simulink model "slb_multirate"  (R2015b)
settings: Solver=FixedStepDiscrete  SolverMode=SingleTasking  StartTime=0.0  StopTime=1  RelTol=1e-3
libraries: simulink x1, dspsigops x1
settings Model: Creator=at-mt  LastModifiedBy=amatsumo
settings DataIOCC: SaveFormat=Array  SignalLoggingSaveFormat=ModelDataLogs  SaveOutput=off  SignalLogging=off  SaveTime=off
settings OptimizationCC: BlockReduction=off  ConditionallyExecuteInputs=off  DefaultParameterBehavior=Inlined  ExpressionDepthLimit=2147483647
settings DebuggingCC: AlgebraicLoopMsg=error  UnderspecifiedInitializationDetection=Classic  MergeDetectMultiDrivingBlocksExec=none  SolverPrmCheckMsg=warning  SingleTaskRateTransMsg=error  FcnCallInpInsideContextMsg=UseLocalSettings  StateNameClashWarn=warning
settings HardwareCC: ProdBitPerPointer=32  ProdLargestAtomicFloat=None  ProdIntDivRoundTo=Undefined  ProdEndianess=Unspecified  ProdWordSize=32  ProdHWDeviceType=ASIC/FPGA->ASIC/FPGA  ProdEqTarget=off
settings SFSimCC: SFSimEcho=off  SimParseCustomCode=off
settings GRTTargetCC: GeneratePreprocessorConditionals=Disable all  CombineOutputUpdateFcns=off  GRTInterface=on
settings ConfigComp: CovModelRefEnable=Off  CovSFcnEnable=off

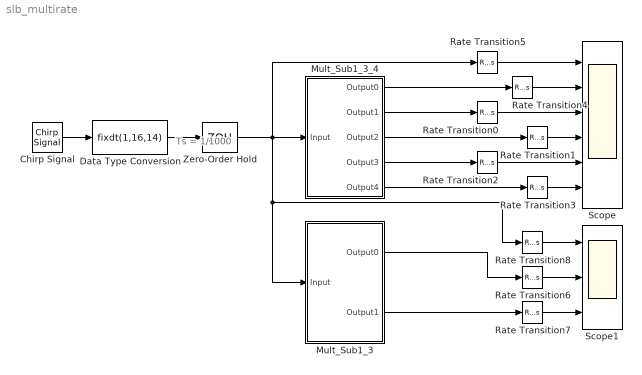
== system slb_multirate ==
  note: Ts = 1/1000
  Chirp Signal : simulink/Sources/Chirp Signal  f1=10  T=1  f2=100
  Data Type Conversion : DataTypeConversion  OutDataTypeStr=fixdt(1,16,14)
  Mult_Sub1_3 : Subsystem  Tag=FilterWizardSubSystem
      settings: ErrorFcn=dspFilterRealizedInBasicElemsAlgLoopErrFcnCallback
  Mult_Sub1_3_4 : Subsystem  Tag=FilterWizardSubSystem
      settings: ErrorFcn=dspFilterRealizedInBasicElemsAlgLoopErrFcnCallback
  Rate Transition{0..8} (9 alike) : RateTransition
  Scope : Scope  NumInputPorts=6
  Scope1 : Scope  NumInputPorts=3
  Zero-Order Hold : ZeroOrderHold  SampleTime=1/1000
  wires:
  Chirp Signal/1 -> Data Type Conversion/1
  Zero-Order Hold/1 -> Mult_Sub1_3_4/1(Input), Rate Transition5/1, Mult_Sub1_3/1(Input), Rate Transition8/1
  Data Type Conversion/1 -> Zero-Order Hold/1
  Mult_Sub1_3_4/1(Output0) -> Rate Transition4/1
  Mult_Sub1_3_4/2(Output1) -> Rate Transition0/1
  Mult_Sub1_3_4/3(Output2) -> Rate Transition1/1
  Rate Transition0/1 -> Scope/3
  Rate Transition1/1 -> Scope/4
  Mult_Sub1_3_4/4(Output3) -> Rate Transition2/1
  Mult_Sub1_3_4/5(Output4) -> Rate Transition3/1
  Rate Transition2/1 -> Scope/5
  Rate Transition3/1 -> Scope/6
  Rate Transition4/1 -> Scope/2
  Rate Transition5/1 -> Scope/1
  Mult_Sub1_3/1(Output0) -> Rate Transition6/1
  Mult_Sub1_3/2(Output1) -> Rate Transition7/1
  Rate Transition6/1 -> Scope1/2
  Rate Transition7/1 -> Scope1/3
  Rate Transition8/1 -> Scope1/1

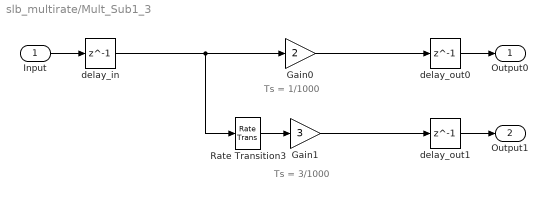
== system slb_multirate/Mult_Sub1_3 ==
  note: Ts = 1/1000
  note: Ts = 3/1000
  Input : Inport
  Gain0 : Gain  Gain=2
  Gain1 : Gain  Gain=3
  Rate Transition3 : RateTransition  OutPortSampleTime=3/1000
  delay_in : Delay  DelayLength=1  InitialCondition=0  InputProcessing=Inherited
  delay_out0 : Delay  DelayLength=1  InitialCondition=0  InputProcessing=Inherited
  delay_out1 : Delay  DelayLength=1  InitialCondition=0  InputProcessing=Inherited
  Output0 : Outport
  Output1 : Outport  Port=2
  wires:
  Gain1/1 -> delay_out1/1
  Gain0/1 -> delay_out0/1
  delay_out1/1 -> Output1/1
  Rate Transition3/1 -> Gain1/1
  delay_out0/1 -> Output0/1
  delay_in/1 -> Gain0/1, Rate Transition3/1
  Input/1 -> delay_in/1

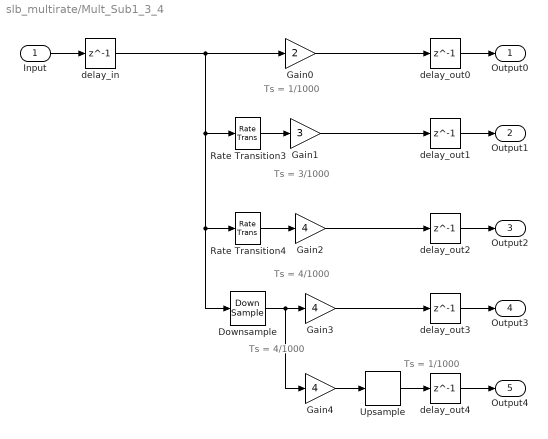
== system slb_multirate/Mult_Sub1_3_4 ==
  note: Ts = 3/1000
  note: Ts = 4/1000
  note: Ts = 1/1000
  note: Ts = 4/1000
  note: Ts = 1/1000
  Input : Inport
  Downsample : DownSample  N=4  RateOptions=Allow multirate processing
  Gain0 : Gain  Gain=2
  Gain1 : Gain  Gain=3
  Gain2 : Gain  Gain=4
  Gain3 : Gain  Gain=4
  Gain4 : Gain  Gain=4
  Rate Transition3 : RateTransition  OutPortSampleTime=3/1000
  Rate Transition4 : RateTransition  OutPortSampleTime=4/1000
  Upsample : dspsigops/Upsample  N=4  phase=0  InputProcessing=Columns as channels (frame based)  RateOptions=Allow multirate processing  ic=0  mode=Unused parameter value
  delay_in : Delay  DelayLength=1  InitialCondition=0  InputProcessing=Inherited
  delay_out{0..4} (5 alike) : Delay  DelayLength=1  InitialCondition=0  InputProcessing=Inherited
  Output0 : Outport
  Output1 : Outport  Port=2
  Output2 : Outport  Port=3
  Output3 : Outport  Port=4
  Output4 : Outport  Port=5
  wires:
  Input/1 -> delay_in/1
  delay_in/1 -> Rate Transition3/1, Rate Transition4/1, Downsample/1, Gain0/1
  delay_out0/1 -> Output0/1
  Rate Transition3/1 -> Gain1/1
  delay_out1/1 -> Output1/1
  Rate Transition4/1 -> Gain2/1
  delay_out2/1 -> Output2/1
  Gain0/1 -> delay_out0/1
  Gain1/1 -> delay_out1/1
  Gain2/1 -> delay_out2/1
  Gain3/1 -> delay_out3/1
  Downsample/1 -> Gain3/1, Gain4/1
  delay_out3/1 -> Output3/1
  Gain4/1 -> Upsample/1
  Upsample/1 -> delay_out4/1
  delay_out4/1 -> Output4/1
